simulink model "tilt_rotor_drone_controller"  (R2020b)
settings: Solver=VariableStepAuto  StartTime=0.0  StopTime=10.0  RelTol=1e-3
values from neighbouring files (symbols this model uses):
  acceleration_bc = zeros(size(trajectory))    [run_sim.m]
  b = 20    [run_sim.m]
  d = 0.5    [run_sim.m]
  gamma = [alpha; beta]    [run_sim.m]
  inertia = [0.0092, 0, 0 ... (first row only)    [run_sim.m]    (also in symbolic_equations.m = [Ixx, 0, 0)
  J_TP = 0.5    [run_sim.m]
  K_attitude = lqr(A_attitude, B_attitude, Q_a, R_a)    [run_sim.m]
  K_gamma = lqr(A_gamma, B_gamma, Q_g, R_g)    [run_sim.m]
  K_gamma_plane = lqr(A_gamma_plane, B_gamma_plane, Q_g_p, R_g_p)    [run_sim.m]
  K_position = lqr(A_position, B_position, Q_p, R_p)    [run_sim.m]
  k_r_attitude = -inv(C_attitude/(A_attitude-B_attitude*K_attitude)*B_attitude)    [run_sim.m]
  k_r_gamma = -inv(C_gamma/(A_gamma-B_gamma*K_gamma)*B_gamma)    [run_sim.m]
  k_r_gamma_plane = -inv(C_gamma_plane/(A_gamma_plane-B_gamma_plane*K_gamma_plane)*B_gamma_plane)    [run_sim.m]
  k_r_position = -inv(C_position/(A_position-B_position*K_position)*B_position)    [run_sim.m]
  k_r_thrust = -inv(C_thrust/(A_thrust-B_thrust*K_thrust)*B_thrust)    [run_sim.m]
  k_r_thrust_plane = -inv(C_thrust_plane/(A_thrust_plane-B_thrust_plane*K_thrust_plane)*B_thrust_plane)    [run_sim.m]
  K_thrust = lqr(A_thrust, B_thrust, Q_t, R_t)    [run_sim.m]
  K_thrust_plane = lqr(A_thrust_plane, B_thrust_plane, Q_t_p, R_t_p)    [run_sim.m]
  l_a = 0    [run_sim.m]
  l_l = 0.154    [run_sim.m]
  l_s = 0.19    [run_sim.m]
  lambda = 0.01    [run_sim.m]
  m = 0.736    [run_sim.m]
  mass = [0.736, 0, 0 ... (first row only)    [run_sim.m]    (also in symbolic_equations.m = m*eye(3))
  rho = 1.1455    [run_sim.m]
  trajectory_time = [1;1.1]    [run_sim.m]
  velocity_bc = zeros(size(trajectory))    [run_sim.m]
  wing_area = 0.000124    [run_sim.m]
undefined symbols (not defined in the file or in its folder): trajectory
libraries: simulink x2, robotcorelib x1
settings Model: OrderedModelArguments=off  Creator=Peter Guglielmino  LastModifiedBy=Peter Guglielmino

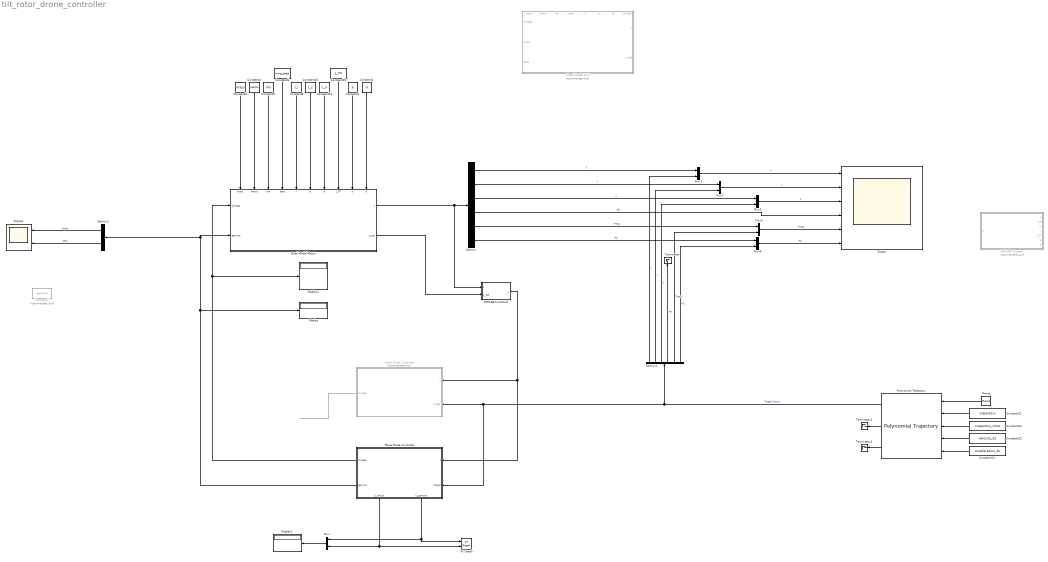
== system tilt_rotor_drone_controller ==
  Constant1 : Constant  Value=b
  Constant10 : Constant  Value=l_s
  Constant13 : Constant  Value=l_a
  Constant2 : Constant  Value=d
  Constant20 : Constant  Value=J_TP
  Constant21 : Constant  Value=trajectory
  Constant22 : Constant  Value=trajectory_time
  Constant23 : Constant  Value=velocity_bc
  Constant24 : Constant  Value=acceleration_bc
  Constant3 : Constant  Value=mass
  Constant4 : Constant  Value=inertia
  Constant5 : Constant  Value=rho
  Constant6 : Constant  Value=wing_area
  Constant7 : Constant  Commented=on  Value=gamma
  Constant8 : Constant  Value=l_l
  Demux : Demux  Outputs=6
  Demux1 : Demux  Outputs=6
  Demux2 : Demux  Outputs=2
  Display : Display
  Display1 : Display
  Display2 : Display
  MATLAB Function : MATLAB Function  Commented=on  TreatAsAtomicUnit=on
  MATLAB Function5 : MATLAB Function  TreatAsAtomicUnit=on
  Mux{,1..5} (6 alike) : Mux  Inputs=2
  Plane Mode Controller : Subsystem
      settings: PortSchema="{\"entries\":[{\"content\":{\"sides\":[{\"content\":{\"connectorIds\":[\"In1\",\"In2\"]},\"type\":\"ConnectorPlacement.EquallySpacedRectSide\",\"uuid\":\"6f4ab3d3-eac6-4fe7-882a-bf2bc23f7ce9\"},{\"content\":{\"connectorIds\":[\"Out1\",\"Out2\"],\"side\":\"RIGHT\"},\"type\":\"ConnectorPlacement.EquallySpacedRectSide\",\"uuid\":\"57ff6c0b-41a8-4a8e-965c-38eb7a1958d7\"},{\"content\":{\"connectorIds\":[],\"side\":\"TOP\"},\"type\":\"ConnectorPlacement.EquallySpacedRectSide\",\"uuid\":\"d6c000f9-9176-43aa-bed6-709b95eb6172\"},{\"content\":{\"connectorIds\":[\"Out3\",\"Out4\"],\"side\":\"BOTTOM\"},\"type\":\"ConnectorPlacement.EquallySpacedRectSide\",\"uuid\":\"a246838b-1dc3-4a22-8023-67a4513b6f5e\"},{\"content\":{\"connectorIds\":[],\"side\":\"HIDDEN\"},\"type\":\"ConnectorPlacement.EquallySpacedRectSide\",\"uuid\":\"9f6f7c1c-aac2-49da-b94c-aa51beb3e11f\"}]},\"type\":\"ConnectorPlacement.EquallySpacedConnector\",\"uuid\":\"622dfaee-5f58-465b-aaa6-50ca0be46197\"}],\"packageUris\":[\"http://schema.mathworks.com/mf0/Connector/R2020b\"],\"version\":\"1.0\"}"
  Polynomial Trajectory : robotcorelib/Polynomial Trajectory  WaypointSource=External  Waypoints=[ 0, 2, 1, 5, 0; -1, 3, 1, 4, 4 ]  TimePoints=[ 0, 1, 2, 3, 4 ]  TimeInterval=[ 1, 4 ]  Method=Quintic Polynomial  ParameterSource=External  VelocityBoundaryCondition=zeros( 2, 5 )  AccelerationBoundaryCondition=zeros( 2, 5 )  SimulateUsing=Interpreted execution
  Quad Mode Controller : Subsystem  Commented=on
  Quad Model F+T : Subsystem  Commented=on
      settings: PortSchema="{\"entries\":[{\"content\":{\"sides\":[{\"content\":{\"connectorIds\":[\"In1\",\"In2\",\"In3\"]},\"type\":\"ConnectorPlacement.EquallySpacedRectSide\",\"uuid\":\"ad073603-3175-40d7-badf-d0e8bcd3f5ed\"},{\"content\":{\"connectorIds\":[\"Out1\",\"Out2\"],\"side\":\"RIGHT\"},\"type\":\"ConnectorPlacement.EquallySpacedRectSide\",\"uuid\":\"d906b516-fe23-4864-8189-1266b65c4bc1\"},{\"content\":{\"connectorIds\":[\"In4\",\"In5\",\"In6\",\"In7\",\"In8\",\"In9\",\"In10\",\"In11\"],\"side\":\"TOP\"},\"type\":\"ConnectorPlacement.EquallySpacedRectSide\",\"uuid\":\"46f69527-661d-433d-ab7a-9aa34cf6966e\"},{\"content\":{\"connectorIds\":[],\"side\":\"HIDDEN\"},\"type\":\"ConnectorPlacement.EquallySpacedRectSide\",\"uuid\":\"d94401f6-fb94-4af8-bf07-62f60ce614d3\"}]},\"type\":\"ConnectorPlacement.EquallySpacedConnector\",\"uuid\":\"9f65350c-1024-4a5e-93be-50f079c0cc08\"}],\"packageUris\":[\"http://schema.mathworks.com/mf0/Connector/R2020b\"],\"version\":\"1.0\"}"
  Quad Model Matrix : Subsystem
      settings: PortSchema="{\"entries\":[{\"content\":{\"sides\":[{\"content\":{\"connectorIds\":[\"In1\",\"In2\"]},\"type\":\"ConnectorPlacement.EquallySpacedRectSide\",\"uuid\":\"7ecde903-2331-4a53-a39c-16ea178ab1ed\"},{\"content\":{\"connectorIds\":[\"Out1\",\"Out2\"],\"side\":\"RIGHT\"},\"type\":\"ConnectorPlacement.EquallySpacedRectSide\",\"uuid\":\"6c8afcf7-f2a3-489f-9b49-f136426d5410\"},{\"content\":{\"connectorIds\":[\"In3\",\"In4\",\"In5\",\"In6\",\"In7\",\"In8\",\"In9\",\"In10\",\"In11\",\"In12\"],\"side\":\"TOP\"},\"type\":\"ConnectorPlacement.EquallySpacedRectSide\",\"uuid\":\"0140aa1b-fbb5-4f49-aa9b-68a16b457c8d\"},{\"content\":{\"connectorIds\":[],\"side\":\"HIDDEN\"},\"type\":\"ConnectorPlacement.EquallySpacedRectSide\",\"uuid\":\"90be69ad-385b-43a9-9593-2c36f7e28e6a\"}]},\"type\":\"ConnectorPlacement.EquallySpacedConnector\",\"uuid\":\"53a680ce-3107-460b-8e4c-bf9b774de8db\"}],\"packageUris\":[\"http://schema.mathworks.com/mf0/Connector/R2020b\"],\"version\":\"1.0\"}"
  Ramp : simulink/Sources/Ramp  slope=0.5  start=0  InitialOutput=0
  Scope : Scope  NumInputPorts=6
  Scope1 : Scope  NumInputPorts=2
  Terminator : Terminator
  Terminator1 : Terminator
  Terminator2 : Terminator
  XY Graph : simulink/Sinks/XY Graph  xmin=-1  xmax=1  ymin=-1  ymax=1  st=-1
  wires:
  Quad Model Matrix/1(s) -> MATLAB Function5/1(s), Demux/1
  Demux/1 -> Mux1/1  "X"
  Demux/2 -> Mux2/1  "Y"
  Demux/3 -> Mux3/1  "Z"
  Demux/4 -> Scope/4  "Phi"
  Demux/6 -> Mux4/1  "Psi"
  Quad Model Matrix/2(s_dot) -> MATLAB Function5/2(s_dot)
  Demux1/6 -> Mux4/2  "Psi"
  Demux1/1 -> Mux1/2  "X"
  Demux1/3 -> Mux3/2  "Z"
  Demux1/2 -> Mux2/2  "Y"
  Mux1/1 -> Scope/1  "X"
  Mux2/1 -> Scope/2  "Y"
  Mux3/1 -> Scope/3  "Z"
  Mux4/1 -> Scope/6  "Psi"
  Constant3/1 -> Quad Model Matrix/3(mass)
  Constant4/1 -> Quad Model Matrix/4(inertia)
  Constant5/1 -> Quad Model Matrix/5(rho)
  Constant6/1 -> Quad Model Matrix/6(area)
  Constant8/1 -> Quad Model Matrix/7(ll)
  Constant10/1 -> Quad Model Matrix/8(ls)
  Constant13/1 -> Quad Model Matrix/9(la)
  Constant20/1 -> Quad Model Matrix/10(J_TP)
  Demux1/5 -> Mux5/2  "Theta"
  Demux/5 -> Mux5/1  "Theta"
  Mux5/1 -> Scope/5  "Theta"
  Constant1/1 -> Quad Model Matrix/11(b)
  Constant2/1 -> Quad Model Matrix/12(d)
  Polynomial Trajectory/1 -> Plane Mode Controller/2(Target), Quad Mode Controller/2(Target), Demux1/1  "Target Vector"
  Ramp/1 -> Polynomial Trajectory/1
  Constant22/1 -> Polynomial Trajectory/3
  Constant21/1 -> Polynomial Trajectory/2
  Constant23/1 -> Polynomial Trajectory/4
  Constant24/1 -> Polynomial Trajectory/5
  Demux1/4 -> Terminator/1  "Phi"
  Polynomial Trajectory/2 -> Terminator1/1
  Polynomial Trajectory/3 -> Terminator2/1
  MATLAB Function5/1(y) -> Plane Mode Controller/1(s), Quad Mode Controller/1(s)
  Demux2/1 -> Scope1/1  "alpha"
  Demux2/2 -> Scope1/2  "beta"
  Plane Mode Controller/2(gamma) -> Demux2/1, Quad Model Matrix/2(gamma), Display/1
  Plane Mode Controller/1(Omega) -> Display2/1, Quad Model Matrix/1(Omega)
  Quad Mode Controller/1(Omega) -> ?
  Plane Mode Controller/3(U_gamma) -> Mux/1, XY Graph/1
  Plane Mode Controller/4(U_thrust) -> XY Graph/2, Mux/2
  Mux/1 -> Display1/1

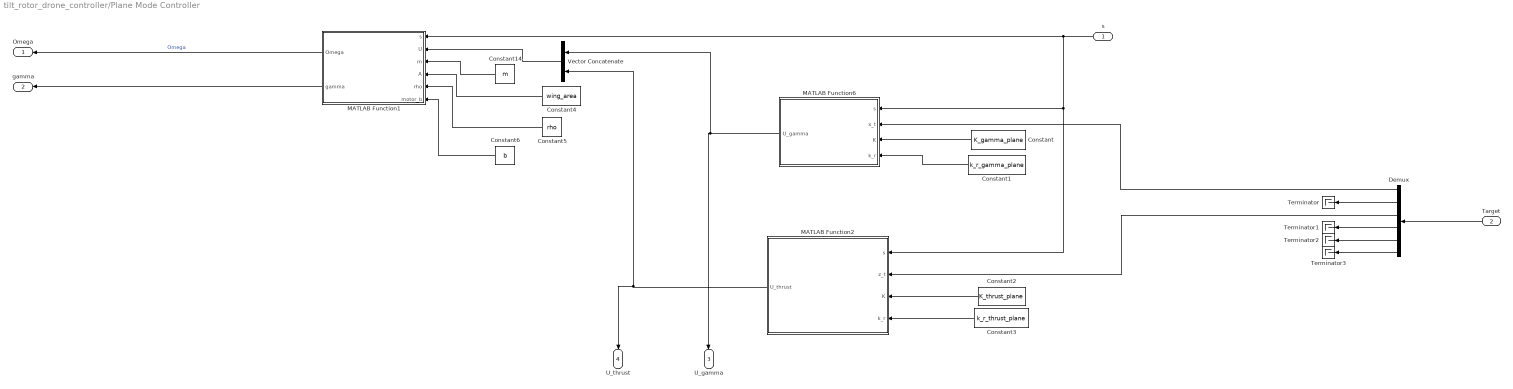
== system tilt_rotor_drone_controller/Plane Mode Controller ==
  s : Inport
  Target : Inport  Port=2
  Constant : Constant  Value=K_gamma_plane
  Constant1 : Constant  Value=k_r_gamma_plane
  Constant14 : Constant  Value=m
  Constant2 : Constant  Value=K_thrust_plane
  Constant3 : Constant  Value=k_r_thrust_plane
  Constant4 : Constant  Value=wing_area
  Constant5 : Constant  Value=rho
  Constant6 : Constant  Value=b
  Demux : Demux  Outputs=6
  MATLAB Function1 : MATLAB Function  TreatAsAtomicUnit=on
  MATLAB Function2 : MATLAB Function  TreatAsAtomicUnit=on
  MATLAB Function6 : MATLAB Function  TreatAsAtomicUnit=on
  Terminator{,1..3} (4 alike) : Terminator
  Vector Concatenate : Concatenate
  Omega : Outport
  gamma : Outport  Port=2
  U_gamma : Outport  Port=3
  U_thrust : Outport  Port=4
  wires:
  Demux/3 -> MATLAB Function2/2(z_t)
  s/1 -> MATLAB Function2/1(s), MATLAB Function6/1(s), MATLAB Function1/1(s)
  MATLAB Function1/1(Omega) -> Omega/1  "Omega"
  Vector Concatenate/1 -> MATLAB Function1/2(U)
  Constant14/1 -> MATLAB Function1/3(m)
  MATLAB Function2/1(U_thrust) -> U_thrust/1, Vector Concatenate/2
  MATLAB Function1/2(gamma) -> gamma/1
  Constant2/1 -> MATLAB Function2/3(K)
  Constant3/1 -> MATLAB Function2/4(k_r)
  Constant/1 -> MATLAB Function6/3(K)
  Constant1/1 -> MATLAB Function6/4(k_r)
  Constant4/1 -> MATLAB Function1/4(A)
  Constant5/1 -> MATLAB Function1/5(rho)
  MATLAB Function6/1(U_gamma) -> Vector Concatenate/1, U_gamma/1
  Constant6/1 -> MATLAB Function1/6(motor_b)
  Target/1 -> Demux/1
  Demux/1 -> MATLAB Function6/2(x_t)
  Demux/2 -> Terminator/1
  Demux/4 -> Terminator1/1
  Demux/5 -> Terminator2/1
  Demux/6 -> Terminator3/1

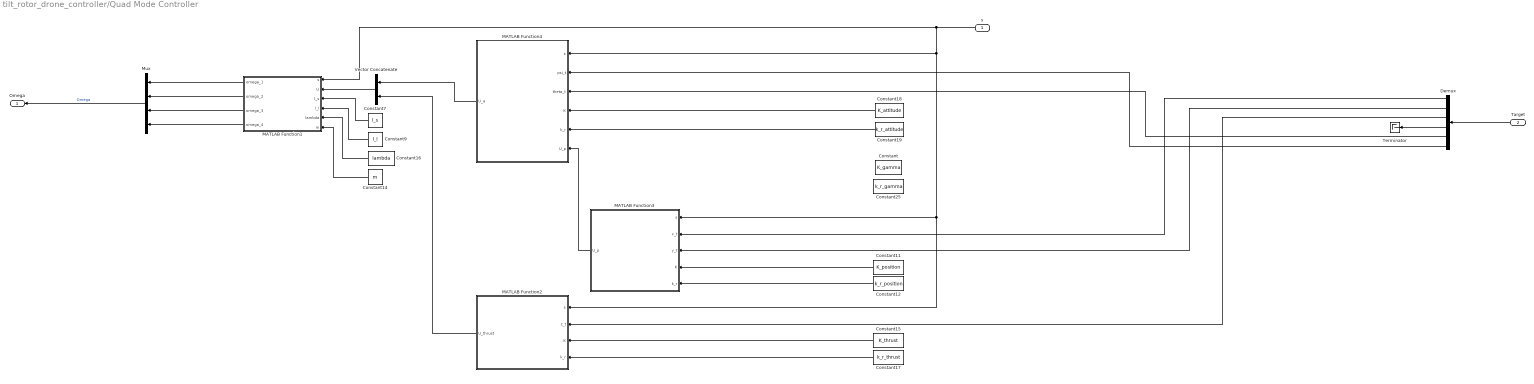
== system tilt_rotor_drone_controller/Quad Mode Controller ==
  s : Inport
  Target : Inport  Port=2
  Constant : Constant  Value=K_gamma
  Constant11 : Constant  Value=K_position
  Constant12 : Constant  Value=k_r_position
  Constant14 : Constant  Value=m
  Constant15 : Constant  Value=K_thrust
  Constant16 : Constant  Value=lambda
  Constant17 : Constant  Value=k_r_thrust
  Constant18 : Constant  Value=K_attitude
  Constant19 : Constant  Value=k_r_attitude
  Constant25 : Constant  Value=k_r_gamma
  Constant7 : Constant  Value=l_s
  Constant9 : Constant  Value=l_l
  Demux : Demux  Outputs=6
  MATLAB Function1 : MATLAB Function  TreatAsAtomicUnit=on
  MATLAB Function2 : MATLAB Function  TreatAsAtomicUnit=on
  MATLAB Function3 : MATLAB Function  TreatAsAtomicUnit=on
  MATLAB Function4 : MATLAB Function  TreatAsAtomicUnit=on
  Mux : Mux
  Terminator : Terminator
  Vector Concatenate : Concatenate
  Omega : Outport
  wires:
  Constant11/1 -> MATLAB Function3/4(K)
  MATLAB Function1/3(omega_3) -> Mux/3
  MATLAB Function1/1(omega_1) -> Mux/1
  s/1 -> MATLAB Function2/1(s), MATLAB Function3/1(s), MATLAB Function4/1(s), MATLAB Function1/1(s)
  MATLAB Function4/1(U_a) -> Vector Concatenate/1
  MATLAB Function1/2(omega_2) -> Mux/2
  MATLAB Function2/1(U_thrust) -> Vector Concatenate/2
  Constant17/1 -> MATLAB Function2/4(k_r)
  Constant16/1 -> MATLAB Function1/5(lambda)
  Constant14/1 -> MATLAB Function1/6(m)
  MATLAB Function1/4(omega_4) -> Mux/4
  MATLAB Function3/1(U_p) -> MATLAB Function4/6(U_p)
  Constant7/1 -> MATLAB Function1/3(l_s)
  Constant9/1 -> MATLAB Function1/4(l_l)
  Demux/6 -> MATLAB Function4/2(psi_t)
  Constant12/1 -> MATLAB Function3/5(k_r)
  Constant19/1 -> MATLAB Function4/5(k_r)
  Vector Concatenate/1 -> MATLAB Function1/2(U)
  Demux/5 -> MATLAB Function4/3(theta_t)
  Constant15/1 -> MATLAB Function2/3(K)
  Constant18/1 -> MATLAB Function4/4(K)
  Demux/1 -> MATLAB Function3/2(x_t)
  Mux/1 -> Omega/1  "Omega"
  Demux/2 -> MATLAB Function3/3(y_t)
  Demux/3 -> MATLAB Function2/2(z_t)
  Demux/4 -> Terminator/1
  Target/1 -> Demux/1

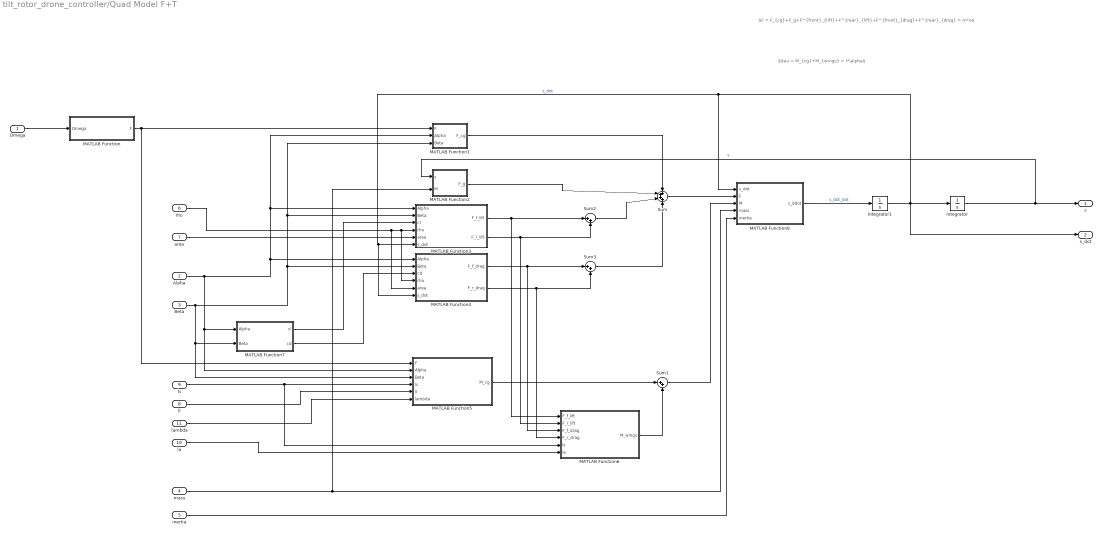
== system tilt_rotor_drone_controller/Quad Model F+T ==
  note: $\tau = M_{cg}+M_{wings} = I*\alpha$
  note: $F = F_{cg}+F_g+F^{front}_{lift}+F^{rear}_{lift}+F^{front}_{drag}+F^{rear}_{drag} = m*a$
  Omega : Inport
  Alpha : Inport  Port=2
  Beta : Inport  Port=3
  mass : Inport  Port=4
  inertia : Inport  Port=5
  rho : Inport  Port=6
  area : Inport  Port=7
  ll : Inport  Port=8
  ls : Inport  Port=9
  la : Inport  Port=10
  lambda : Inport  Port=11
  Integrator : Integrator
  Integrator1 : Integrator
  MATLAB Function : MATLAB Function  TreatAsAtomicUnit=on
  MATLAB Function1 : MATLAB Function  TreatAsAtomicUnit=on
  MATLAB Function2 : MATLAB Function  TreatAsAtomicUnit=on
  MATLAB Function3 : MATLAB Function  TreatAsAtomicUnit=on
  MATLAB Function4 : MATLAB Function  TreatAsAtomicUnit=on
  MATLAB Function5 : MATLAB Function  TreatAsAtomicUnit=on
  MATLAB Function6 : MATLAB Function  TreatAsAtomicUnit=on
  MATLAB Function7 : MATLAB Function  TreatAsAtomicUnit=on
  MATLAB Function8 : MATLAB Function  TreatAsAtomicUnit=on
  Sum : Sum  Inputs=++++
  Sum1 : Sum  Inputs=|++
  Sum2 : Sum  Inputs=|++
  Sum3 : Sum  Inputs=|++
  s : Outport
  s_dot : Outport  Port=2
  wires:
  MATLAB Function/1(F) -> MATLAB Function1/1(F), MATLAB Function5/1(F)
  MATLAB Function7/2(cd) -> MATLAB Function4/3(cd)
  MATLAB Function7/1(cl) -> MATLAB Function3/3(cl)
  inertia/1 -> MATLAB Function8/5(inertia)
  mass/1 -> MATLAB Function2/2(M), MATLAB Function8/4(mass)
  Sum1/1 -> MATLAB Function8/3(M)
  Sum/1 -> MATLAB Function8/2(F)
  la/1 -> MATLAB Function6/6(la)
  MATLAB Function4/2(F_r_drag) -> Sum3/2, MATLAB Function6/4(F_r_drag)
  MATLAB Function4/1(F_f_drag) -> Sum3/1, MATLAB Function6/3(F_f_drag)
  MATLAB Function3/2(F_r_lift) -> Sum2/2, MATLAB Function6/2(F_r_lift)
  MATLAB Function3/1(F_f_lift) -> Sum2/1, MATLAB Function6/1(F_f_lift)
  Sum3/1 -> Sum/4
  Sum2/1 -> Sum/3
  lambda/1 -> MATLAB Function5/6(lambda)
  ll/1 -> MATLAB Function5/5(ll)
  ls/1 -> MATLAB Function5/4(ls), MATLAB Function6/5(ls)
  area/1 -> MATLAB Function3/5(area)
  rho/1 -> MATLAB Function3/4(rho), MATLAB Function4/4(rho), MATLAB Function4/5(area)
  Beta/1 -> MATLAB Function3/2(Beta), MATLAB Function1/3(Beta), MATLAB Function4/2(Beta), MATLAB Function7/2(Beta), MATLAB Function5/3(Beta)
  Alpha/1 -> MATLAB Function4/1(Alpha), MATLAB Function3/1(Alpha), MATLAB Function1/2(Alpha), MATLAB Function7/1(Alpha), MATLAB Function5/2(Alpha)
  MATLAB Function8/1(s_ddot) -> Integrator1/1  "s_dot_dot"
  MATLAB Function6/1(M_wings) -> Sum1/2
  MATLAB Function5/1(M_cg) -> Sum1/1
  MATLAB Function2/1(F_g) -> Sum/2
  MATLAB Function1/1(F_cg) -> Sum/1
  Omega/1 -> MATLAB Function/1(Omega)
  Integrator1/1 -> s_dot/1, Integrator/1, MATLAB Function8/1(s_dot), MATLAB Function3/6(s_dot), MATLAB Function4/6(s_dot)  "s_dot"
  Integrator/1 -> s/1, MATLAB Function2/1(s)  "s"

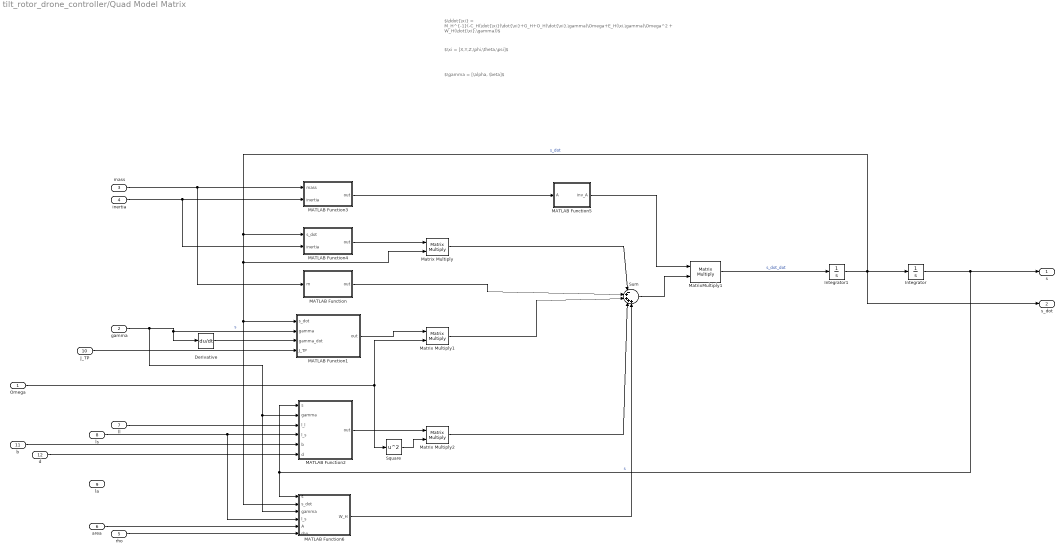
== system tilt_rotor_drone_controller/Quad Model Matrix ==
  note: $\ddot{\xi} = M_H^{-1}(-C_H(\dot{\xi})\dot{\xi}+G_H+O_H(\dot{\xi},\gamma)\Omega+E_H(\xi,\gamma)\Omega^2 + W_H(\dot{\xi},\gamma))$
  note: $\xi = [X,Y,Z,\phi,\theta,\psi]$
  note: $\gamma = [\alpha, \beta]$
  Omega : Inport  PortDimensions=[4,1]
  gamma : Inport  Port=2  PortDimensions=[2 1]
  mass : Inport  Port=3
  inertia : Inport  Port=4
  rho : Inport  Port=5
  area : Inport  Port=6
  ll : Inport  Port=7
  ls : Inport  Port=8
  la : Inport  Port=9
  J_TP : Inport  Port=10
  b : Inport  Port=11
  d : Inport  Port=12
  Derivative : Derivative
  Integrator : Integrator
  Integrator1 : Integrator
  MATLAB Function : MATLAB Function  TreatAsAtomicUnit=on
  MATLAB Function1 : MATLAB Function  TreatAsAtomicUnit=on
  MATLAB Function2 : MATLAB Function  TreatAsAtomicUnit=on
  MATLAB Function3 : MATLAB Function  TreatAsAtomicUnit=on
  MATLAB Function4 : MATLAB Function  TreatAsAtomicUnit=on
  MATLAB Function5 : MATLAB Function  TreatAsAtomicUnit=on
  MATLAB Function6 : MATLAB Function  TreatAsAtomicUnit=on
  Matrix Multiply : Product  Multiplication=Matrix(*)
  Matrix Multiply1 : Product  Multiplication=Matrix(*)
  Matrix Multiply2 : Product  Multiplication=Matrix(*)
  MatrixMultiply1 : Product  Multiplication=Matrix(*)
  Square : Math  Operator=square  SaturateOnIntegerOverflow=on
  Sum : Sum  Inputs=|-++++
  s : Outport
  s_dot : Outport  Port=2
  wires:
  Integrator/1 -> MATLAB Function2/1(s), MATLAB Function6/1(s), s/1  "s"
  Integrator1/1 -> s_dot/1, MATLAB Function4/1(s_dot), Matrix Multiply/2, MATLAB Function6/2(s_dot), MATLAB Function1/1(s_dot), Integrator/1  "s_dot"
  MatrixMultiply1/1 -> Integrator1/1  "s_dot_dot"
  MATLAB Function/1(out) -> Sum/2
  Matrix Multiply/1 -> Sum/1
  Sum/1 -> MatrixMultiply1/2
  MATLAB Function1/1(out) -> Matrix Multiply1/1
  Matrix Multiply1/1 -> Sum/3
  MATLAB Function2/1(out) -> Matrix Multiply2/1
  Matrix Multiply2/1 -> Sum/4
  mass/1 -> MATLAB Function/1(m), MATLAB Function3/1(mass)
  inertia/1 -> MATLAB Function4/2(inertia), MATLAB Function3/2(inertia)
  ll/1 -> MATLAB Function2/3(l_l)
  ls/1 -> MATLAB Function6/4(l_s), MATLAB Function2/4(l_s)
  b/1 -> MATLAB Function2/5(b)
  d/1 -> MATLAB Function2/6(d)
  J_TP/1 -> MATLAB Function1/4(J_TP)
  MATLAB Function4/1(out) -> Matrix Multiply/1
  Square/1 -> Matrix Multiply2/2
  Omega/1 -> Matrix Multiply1/2, Square/1
  MATLAB Function3/1(out) -> MATLAB Function5/1(A)
  MATLAB Function5/1(inv_A) -> MatrixMultiply1/1
  gamma/1 -> MATLAB Function6/3(gamma), MATLAB Function2/2(gamma), MATLAB Function1/2(gamma), Derivative/1  "s"
  area/1 -> MATLAB Function6/5(A)
  rho/1 -> MATLAB Function6/6(rho)
  MATLAB Function6/1(W_H) -> Sum/5
  Derivative/1 -> MATLAB Function1/3(gamma_dot)

== matlab function tilt_rotor_drone_controller/Quad Mode Controller/MATLAB Function2 ==
  data: s input; z_t input; K input size=[1 2]; k_r input size=1; U_thrust output
function U_thrust = thrust_control(s, z_t, K, k_r)

% s = [x, dx, y, dy, z, dz, phi, p, theta, q, psi, r]

x = s(5:6);
x_d = [z_t; 0];

C = [1,0];
r = C*x_d;

U_thrust = -K*x + k_r*r;

== matlab function tilt_rotor_drone_controller/Quad Mode Controller/MATLAB Function3 ==
  data: s input; U_p output; x_t input; y_t input; K input size=[2 4]; k_r input size=[2 2]
function U_p = position_control(s, x_t, y_t, K, k_r)

% s = [x, dx, y, dy, z, dz, phi, p, theta, q, psi, r]

x = s(1:4);
x_d = [x_t;0;y_t;0];
  
C = [1,0,0,0;
     0,0,1,0];

r = C*x_d;
U_p = -K*x + k_r*r;

== matlab function tilt_rotor_drone_controller/Quad Mode Controller/MATLAB Function4 ==
  data: s input; psi_t input; theta_t input; U_a output; K input size=[3 6]; k_r input size=[3 3]; U_p input
function U_a  = attitude_control(s, psi_t, theta_t, K, k_r, U_p)

% s = [x, dx, y, dy, z, dz, !phi, p, theta, q, psi, r!]
% U_p = [U_x, U_y]
% U_x = (cos(phi)*sin(theta)*cos(psi) + sin(phi)*sin(psi))/(cos(phi)*cos(theta))
% U_y = (cos(phi)*sin(theta)*sin(psi) - sin(phi)*cos(psi))/(cos(phi)*cos(theta))
% theta = atan2(U_y + U_x*tan(psi),sin(psi)-cos(psi)^2)
% phi = atan2(U_x*cos(theta)-sin(theta)*cos(psi),sin(psi))

% alpha = 0;
% beta = 0;


x = s(7:12);

U_x = U_p(1);
U_y = U_p(2);

psi = x(5);
Kappa = U_x^2 + U_y^2;

if (U_x^2 + U_y^2) == 0
    phi = 0;
else
    phi = asin(sqrt(Kappa/((1+Kappa)*(U_x^2+U_y^2))) * (U_x*sin(psi) - U_y*cos(psi)));
end

s = sign(U_y*sin(psi) + U_x*cos(psi));
if abs(1/(cos(phi)*sqrt(1+Kappa))) > 1
    theta = s*acos(sign(1/(cos(phi)*sqrt(1+Kappa))));
else
    theta = s*acos(1/(cos(phi)*sqrt(1+Kappa)));
end

x_d = [phi; 0; theta + theta_t; 0; psi_t; 0];
 
C = [1,0,0,0,0,0;
     0,0,1,0,0,0;
     0,0,0,0,1,0];
 
r = C*x_d;
U_a = -K*x + k_r*r;

== matlab function tilt_rotor_drone_controller/MATLAB Function5 ==
  data: s input; y output; s_dot input
function y = mixer(s, s_dot)

x = [s(1);s_dot(1);s(2);s_dot(2);s(3);s_dot(3);s(4);s_dot(4);s(5);s_dot(5);s(6);s_dot(6)];

y = x;

== matlab function tilt_rotor_drone_controller/Quad Model Matrix/MATLAB Function6 ==
  data: s input size=[6 1]; s_dot input size=[6 1]; W_H output size=[6 1]; gamma input size=[2 1]; l_s input size=1; A input size=1; rho input size=1
function W_H = W_H(s, s_dot, gamma, l_s, A, rho)
% s_dot = [dx, dy, dz, p, q, r]

v = [s_dot(1); 0; s_dot(3)]; % wind velocity ignoring y
wind_vel = norm(v)*v;

alpha = gamma(1);
beta = gamma(2);

phi = s(4);
theta = s(5);
psi = s(6);

alpha_matrix = [cos(alpha),  0, sin(alpha);
                    0,       1,      0;
                -sin(alpha), 0, cos(alpha)];
    
beta_matrix = [cos(beta),  0, sin(beta);
                    0,     1,     0;
               -sin(beta), 0, cos(beta)];

alpha_vector = [-sin(alpha); 0; -cos(alpha)];
beta_vector = [-sin(beta); 0; -cos(beta)];


R = [cos(psi)*cos(theta), -sin(psi)*cos(phi) + cos(psi)*sin(theta)*sin(phi), sin(psi)*sin(phi) + cos(psi)*sin(theta)*cos(phi);
     sin(psi)*cos(theta), cos(psi)*cos(phi) + sin(psi)*sin(theta)*sin(phi), -cos(psi)*sin(phi) + sin(psi)*sin(theta)*cos(phi);
     -sin(theta), cos(theta)*sin(phi), cos(theta)*cos(phi)];
 
T = [R, zeros(3,3);
     zeros(3,3), eye(3)];

if norm(wind_vel) ~= 0
    attack_angle_front = acosd(dot(wind_vel,alpha_vector)/(norm(wind_vel)*norm(alpha_vector)));
    attack_angle_back  = acosd(dot(wind_vel,beta_vector)/(norm(wind_vel)*norm(beta_vector)));
    
    c_la = getLiftCoef(attack_angle_front);
    c_lb = getLiftCoef(attack_angle_back);
    c_da = getDragCoef(attack_angle_front);
    c_db = getDragCoef(attack_angle_back);
else
    c_la = 0;
    c_lb = 0;
    c_da = 0;
    c_db = 0;
end

L_pba = alpha_matrix * [1;0;0] * c_la*rho*A * norm(wind_vel);
L_pbb = beta_matrix * [1;0;0] * c_lb*rho*A * norm(wind_vel);
L_pb = L_pba + L_pbb;
L_tb = cross([l_s;0;0], L_pba) + cross([-l_s;0;0], L_pbb);

L_H = T*[L_pb;
         L_tb];
     
D_pba = alpha_matrix * [0;0;1] * c_da*rho*A * norm(wind_vel);
D_pbb = beta_matrix * [0;0;1] * c_db*rho*A * norm(wind_vel);
D_pb = D_pba + D_pbb;
D_tb = cross([l_s;0;0], D_pba) + cross([-l_s;0;0], D_pbb);

D_H = T*[D_pb;
         D_tb];

W_H = L_H + D_H;
end


function c_l = getLiftCoef(x)
    if x > 0 && x < 80
        c_l = -3E-10*x^6 + 7E-08*x^5 - 6E-06*x^4 + 0.0002*x^3 - 0.0042*x^2 + 0.0495*x + 0.0485;
    else
        c_l = 0;
    end
end

function c_d = getDragCoef(x)
    if x > 0 && x < 80
        c_d = 4E-09*x^5 - 8E-07*x^4 + 4E-05*x^3 - 0.0006*x^2 + 0.004*x + 0.0403;
    else
        c_d = 0;
    end
end

== matlab function tilt_rotor_drone_controller/Plane Mode Controller/MATLAB Function1 ==
  data: s input; U input size=[2 1]; Omega output size=[4 1]; m input; gamma output; A input; rho input; motor_b input
function [Omega, gamma]= U_to_Omega(s, U, m, A, rho, motor_b)
% s = [x, dx, y, dy, z, dz, phi, p, theta, q, psi, r]
% U = [U_G, U_T]

U_G = U(1);
U_T = U(2);

g = 9.8;

control_vector = [U_G; U_T];

if norm(control_vector) == 0
    control_angle = 0;
else
    control_angle = -pi/2 + atan2(-control_vector(2),control_vector(1));
end

thrust_value = norm(control_vector);

control_angle = min(max(control_angle, -pi/2), pi/2);

% v = [s(2); 0; s(6)]; % wind velocity ignoring y
% v_w = norm(v)*v;
% 
% alpha_old = -pi/3;
% 
% alpha_vector = [-sin(alpha_old); 0; -cos(alpha_old)];
% 
% phi = s(7);
% theta = s(9);
% psi = s(11);
% 
% K1 = cos(psi)*cos(theta);
% K2 = sin(phi)*sin(psi) + cos(phi)*cos(psi)*sin(theta);
% 
% K3 = sin(theta);
% K4 = cos(phi)*cos(theta);
% 
% if norm(v_w) ~= 0
%     attack_angle_front = acosd(dot(v_w,alpha_vector)/(norm(v_w)*norm(alpha_vector)));
%     
%     c_la = getLiftCoef(attack_angle_front);
%     c_da = getDragCoef(attack_angle_front);
% else
%     c_la = 0;
%     c_da = 0;
% end

% a = K4;
% b = K3;
% c = -m*(U_G - g)/(2*A*rho*norm(v_w)*c_la);
% if c == Inf
%     alpha = alpha_old;
% else
%     d = sqrt(-1*(c^2 - b^2 - a^2));
%     alpha = atan((b*d + a*c)/(b*c - a*d));
% end

% if norm(v_w) ~= 0
%     alpha = alpha_old;
% else
% %     alpha = asin(-m*(U_G - g)/(2*A*rho*norm(v_w)*c_la));
%     alpha = alpha_old;
% end

% omega_1_sqr = -U_T*m/(8*motor_b*(sin(alpha)*K1 + cos(alpha)*K2));
% omega_1_sqr = -((U_T*m + 2*A*rho*norm(v_w)*c_la*cos(alpha) - 2*A*rho*norm(v_w)*c_da*sin(alpha))/(8*motor_b));

alpha = control_angle;
omega_1_sqr = thrust_value;

if (omega_1_sqr > 0)
    omega_1 = sqrt(omega_1_sqr);
else
    omega_1 = 0;
end

gamma = [alpha; alpha];
Omega = [omega_1; omega_1; omega_1; omega_1];

end

function c_l = getLiftCoef(x)
    c_l = -3E-10*x^6 + 7E-08*x^5 - 6E-06*x^4 + 0.0002*x^3 - 0.0042*x^2 + 0.0495*x + 0.0485;
end

function c_d = getDragCoef(x)
    c_d = 4E-09*x^5 - 8E-07*x^4 + 4E-05*x^3 - 0.0006*x^2 + 0.004*x + 0.0403;
end

== matlab function tilt_rotor_drone_controller/Quad Model F+T/MATLAB Function ==
  data: Omega input; F output size=[4 1]
function F = Omega_to_F(Omega)

F = eye(4)*Omega;

== matlab function tilt_rotor_drone_controller/Quad Model F+T/MATLAB Function1 ==
  data: F input; F_cg output; Alpha input; Beta input
function F_cg = F_cg(F, Alpha, Beta)
% Force generated from the rotors

F_cg = [-sin(Alpha)*(F(1)+F(2)) - sin(Beta)*(F(3)+F(4));
                            0;
     -cos(Alpha)*(F(1)+F(2)) - cos(Beta)*(F(3)+F(4))];

== matlab function tilt_rotor_drone_controller/Quad Model F+T/MATLAB Function2 ==
  data: s input; M input; F_g output
function F_g = F_g(s, M)
% s = [x, y, z, phi, theta, psi]
theta = s(5);
phi = s(4);
g = 9.8;

rotation = [-sin(theta);
            sin(phi)*cos(theta);
            cos(phi)*cos(theta)];

F_g = M*rotation*g;

== matlab function tilt_rotor_drone_controller/Quad Model F+T/MATLAB Function3 ==
  data: F_f_lift output; Alpha input; Beta input; cl input; rho input; area input; s_dot input; F_r_lift output
function [F_f_lift, F_r_lift] = F_lift(Alpha, Beta, cl, rho, area, s_dot)
% s_dot = [dx, dy, dz, p, q, r]

Ry_a = [cos(Alpha), 0, sin(Alpha);
             0,     1,      0;
        -sin(Alpha), 0, cos(Alpha)];

Ry_b = [cos(Beta), 0, sin(Beta);
             0,     1,      0;
        -sin(Beta), 0, cos(Beta)];

w_hat = [0;0;-1];

v = [s_dot(1);s_dot(2);s_dot(3)];
v_f = dot(Ry_a * w_hat,v);
v_r = dot(Ry_b * w_hat,v);


F_f_lift = Ry_a * [-2*(1/2)*cl(1)*rho*area*v_f^2;0;0];
F_r_lift = Ry_b * [-2*(1/2)*cl(2)*rho*area*v_r^2;0;0];

== matlab function tilt_rotor_drone_controller/Quad Model Matrix/MATLAB Function1 ==
  data: s_dot input; gamma input size=[2 1]; out output size=[6,4]; gamma_dot input size=[2 1]; J_TP input
function out = O_H(s_dot, gamma, gamma_dot, J_TP)

w_b = s_dot(4:6);

alpha = gamma_dot(1);
beta = gamma(2);

alpha_dot = gamma_dot(1);
beta_dot = gamma_dot(2);

alpha_vector = [-sin(alpha); 0; -cos(alpha)];
beta_vector = [-sin(beta); 0; -cos(beta)];

a_vector = cross(w_b, alpha_vector) + cross([0; alpha_dot; 0], alpha_vector);
b_vector = cross(w_b, beta_vector) + cross([0; beta_dot; 0], beta_vector);
four_vector = [a_vector, -a_vector, -b_vector, b_vector];
O_H = [zeros(3,4);  four_vector];

out = J_TP * O_H;

== matlab function tilt_rotor_drone_controller/Quad Model F+T/MATLAB Function4 ==
  data: Alpha input; Beta input; F_f_drag output; cd input; rho input; area input; s_dot input; F_r_drag output
function [F_f_drag, F_r_drag] = F_drag(Alpha, Beta, cd, rho, area, s_dot)
% s_dot = [dx, dy, dz, p, q, r]

Ry_a = [cos(Alpha), 0, sin(Alpha);
             0,     1,      0;
        -sin(Alpha), 0, cos(Alpha)];

Ry_b = [cos(Beta), 0, sin(Beta);
             0,     1,      0;
        -sin(Beta), 0, cos(Beta)];

w_hat = [0;0;-1];

v = [s_dot(1);s_dot(2);s_dot(3)];
v_f = dot(Ry_a * w_hat,v);
v_r = dot(Ry_b * w_hat,v);


F_f_drag = Ry_a * [0;0;2*(1/2)*cd(1)*rho*area*v_f^2];
F_r_drag = Ry_b * [0;0;2*(1/2)*cd(2)*rho*area*v_r^2];

== matlab function tilt_rotor_drone_controller/Quad Model F+T/MATLAB Function5 ==
  data: F input; M_cg output; Alpha input; Beta input; ls input; ll input; lambda input
function M_cg = M_cg(F, Alpha, Beta, ls, ll, lambda)

Ry_a = [cos(Alpha), 0, sin(Alpha);
            0,     1,      0;
        -sin(Alpha), 0, cos(Alpha)];

Ry_b = [cos(Beta), 0, sin(Beta);
            0,     1,      0;
        -sin(Beta), 0, cos(Beta)];

moment_arm_f = [ls, -ls;
                ll, ll;
                lambda, -lambda];
            
moment_arm_r = [ls, -ls;
                -ll, -ll;
                -lambda, lambda];

M_cg = Ry_a * moment_arm_f * [F(1); F(2)] + Ry_b * moment_arm_r * [F(3); F(4)];

== matlab function tilt_rotor_drone_controller/Quad Model F+T/MATLAB Function6 ==
  data: F_f_lift input; M_wings output; F_r_lift input; F_f_drag input; F_r_drag input; ls input; la input
function M_wings = M_wings(F_f_lift, F_r_lift, F_f_drag, F_r_drag, ls, la)

moment_arm_f = [0, 0, 0;
              -la, 0, -ls;
              0, 0, 0];

moment_arm_r = [0, 0, 0;
              -la, 0, ls;
              0, 0, 0];         
          
M_wings = moment_arm_f*(F_f_lift + F_f_drag) + moment_arm_r*(F_r_lift + F_r_drag);

== matlab function tilt_rotor_drone_controller/Quad Model F+T/MATLAB Function7 ==
  data: Alpha input; cl output; Beta input; cd output
function [cl,cd] = lift_and_drag(Alpha, Beta)

% cl = [cl_f; cl_r]
% cd = [cd_f; cd_r]

cl = [Alpha; Alpha];
cd = [Beta; Beta];

== matlab function tilt_rotor_drone_controller/Quad Model F+T/MATLAB Function8 ==
  data: s_dot input; s_ddot output size=[6 1]; F input; M input; mass input; inertia input
function s_ddot = s_ddot(s_dot, F, M, mass, inertia)
% s_dot = [dx, dy, dz, p, q, r]
% 
% R_x = [1, 0, 0;
%      0, cos(s(7)), -sin(s(7));
%      0, sin(s(7)), cos(s(7))];
% 
% R_y = [cos(s(9)), 0, sin(s(9));
%          0,   1,    0;
%        -sin(s(9)), 0, cos(s(9))];
%   
% R_z = [cos(s(11)), -sin(s(11)), 0;
%        sin(s(11)), cos(s(11)),  0;
%          0,     0,    1];
% 
% T = R_x*R_y*R_z;
% 
% E = [1, 0, -sin(theta);
%      0, cos(theta), sin(phi)*cos(theta);
%      0, -sin(theta), cos(phi)*cos(theta)];

V_b = [s_dot(1);s_dot(2);s_dot(3)];
w_b = [s_dot(4);s_dot(5);s_dot(6)]; 


% P_dot = T\V_b;
V_dot = mass\(F-cross(w_b, mass*V_b));
% Q_dot = E\w_b;
w_dot = inertia\(M-cross(w_b, inertia*w_b));



s_ddot = [V_dot(1); V_dot(2); V_dot(3); w_dot(1); w_dot(2); w_dot(3)];

== matlab function tilt_rotor_drone_controller/Plane Mode Controller/MATLAB Function2 ==
  data: s input; z_t input; K input size=[1 2]; k_r input size=1; U_thrust output
function U_thrust = thrust_control(s, z_t, K, k_r)
% s = [x, dx, y, dy, z, dz, phi, p, theta, q, psi, r]

x = s(5:6);
x_d = [z_t; 0];

C = [1, 0];
r = C*x_d;

U_thrust = -K*x + k_r*r;

== matlab function tilt_rotor_drone_controller/Plane Mode Controller/MATLAB Function6 ==
  data: s input size=[12 1]; x_t input; U_gamma output; K input size=[1 2]; k_r input size=1
function U_gamma = gamma_control(s, x_t, K, k_r)
% s = [x, dx, y, dy, z, dz, phi, p, theta, q, psi, r]
% gamma = [I_alpha, alpha, I_beta, beta]

x = s(1:2);
x_d = [x_t; 0];

C = [1, 0];
r = C*x_d;

U_gamma = -K*x + k_r*r;

== matlab function tilt_rotor_drone_controller/Quad Model Matrix/MATLAB Function ==
  data: m input; out output
function out = G_H(m)

G = m*[0;0;9.8];

out = [G;0;0;0];

== matlab function tilt_rotor_drone_controller/Quad Model Matrix/MATLAB Function2 ==
  data: s input; out output; gamma input size=[2 1]; l_l input; l_s input; b input; d input
function out = E_H(s, gamma, l_l, l_s, b, d)


phi = s(4);
theta = s(5);
psi = s(6);

alpha = gamma(1);
beta = gamma(2);

R = [cos(psi)*cos(theta), -sin(psi)*cos(phi) + cos(psi)*sin(theta)*sin(phi), sin(psi)*sin(phi) + cos(psi)*sin(theta)*cos(phi);
     sin(psi)*cos(theta), cos(psi)*cos(phi) + sin(psi)*sin(theta)*sin(phi), -cos(psi)*sin(phi) + sin(psi)*sin(theta)*cos(phi);
     -sin(theta), cos(theta)*sin(phi), cos(theta)*cos(phi)];

E_B = [-b*sin(alpha), -b*sin(alpha), -b*sin(beta), -b*sin(beta);
        0,0,0,0;
        -b*cos(alpha), -b*cos(alpha), -b*cos(beta), -b*cos(beta);
        b*l_l*cos(alpha) + d*sin(alpha), -1*(b*l_l*cos(alpha) + d*sin(alpha)), b*l_l*cos(beta) - d*sin(beta), -1*(b*l_l*cos(beta) - d*sin(beta));
        b*l_s*cos(alpha), b*l_s*cos(alpha), -1*(b*l_s)*cos(beta), -1*(b*l_s)*cos(beta);
        -b*l_l*sin(alpha) + d*cos(alpha), b*l_l*sin(alpha) - d*cos(alpha), -b*l_l*sin(beta) - d*cos(beta), b*l_l*sin(beta) + d*cos(beta)];
       
T = [R, zeros(3,3);
    zeros(3,3), eye(3)];


out = T*E_B;

== matlab function tilt_rotor_drone_controller/Quad Model Matrix/MATLAB Function3 ==
  data: mass input; out output; inertia input
function out = M_H(mass, inertia)

M = mass * eye(3);

out = [M, zeros(3,3);
    zeros(3,3), inertia];

== matlab function tilt_rotor_drone_controller/Quad Model Matrix/MATLAB Function4 ==
  data: s_dot input; out output size=[6,6]; inertia input
function out = C_H(s_dot, inertia)

skew = inertia*s_dot(4:6);

out = [zeros(3,3), zeros(3,3);
       zeros(1,3), 0, -skew(3), skew(2);
       zeros(1,3), skew(3), 0, -skew(1);
       zeros(1,3), -skew(2), skew(1), 0];

== matlab function tilt_rotor_drone_controller/Quad Model Matrix/MATLAB Function5 ==
  data: A input; inv_A output
function inv_A = m_inverse(A)
inv_A = inv(A);

== matlab function tilt_rotor_drone_controller/MATLAB Function ==
  data: s input; U output; s_d input; m input; I input; J_TP input; Q input; R input
function U = LQR(s, s_d, m, I, J_TP, Q, R)
% s_d = [x_d, 0, y_d, 0, z_d, 0, 0, 0, 0, 0, psi_d, 0]

coder.extrinsic('lqr');

Ix = I(1);
Iy = I(5);
Iz = I(9);

x = s(1);
y = s(3);
z = s(5);
psi = s(11);

theta = 0;
phi = 0;
q = 0;
r = 0;
p = 0;

g = 9.8;

U1 = m*g;
U2 = 0;
U3 = 0;
U4 = 0;
Omega = 0;

U_ss = [U1; U2; U3; U4; Omega];

A = [ 0, 1, 0, 0, 0, 0,                                                          0,       0,                                   0,        0,                                                         0, 0;
    0, 0, 0, 0, 0, 0,  (U1*(cos(phi)*sin(psi) - cos(psi)*sin(phi)*sin(theta)))/5,       0, (U1*cos(phi)*cos(psi)*cos(theta))/5,        0, (U1*(cos(psi)*sin(phi) - cos(phi)*sin(psi)*sin(theta)))/5, 0;
    0, 0, 0, 1, 0, 0,                                                          0,       0,                                   0,        0,                                                         0, 0;
    0, 0, 0, 0, 0, 0, -(U1*(cos(phi)*cos(psi) + sin(phi)*sin(psi)*sin(theta)))/5,       0, (U1*cos(phi)*cos(theta)*sin(psi))/5,        0, (U1*(sin(phi)*sin(psi) + cos(phi)*cos(psi)*sin(theta)))/5, 0;
    0, 0, 0, 0, 0, 1,                                                          0,       0,                                   0,        0,                                                         0, 0;
    0, 0, 0, 0, 0, 0,                                -(U1*cos(theta)*sin(phi))/5,       0,         -(U1*cos(phi)*sin(theta))/5,        0,                                                         0, 0;
    0, 0, 0, 0, 0, 0,                                                          0,       1,                                   0,        0,                                                         0, 0;
    0, 0, 0, 0, 0, 0,                                                          0,       0,                                   0, -5*Omega,                                                         0, 0;
    0, 0, 0, 0, 0, 0,                                                          0,       0,                                   0,        1,                                                         0, 0;
    0, 0, 0, 0, 0, 0,                                                          0, 5*Omega,                                   0,        0,                                                         0, 0;
    0, 0, 0, 0, 0, 0,                                                          0,       0,                                   0,        0,                                                         0, 1;
    0, 0, 0, 0, 0, 0,                                                          0,       0,                                   0,        0,                                                         0, 0];

% a1 = ((Iy-Iz)/Ix)*r - J_TP/Ix*Omega;
% a2 = ((Iz-Ix)/Iy)*r + J_TP/Iy*Omega;
% a3 = ((Ix-Iy)/Iz)*q;
% 
% A = [0,1,0,0,0,0,0,0,0,0,0,0;
%      0,0,0,0,0,0,0,0,0,0,0,0;
%      0,0,0,1,0,0,0,0,0,0,0,0;
%      0,0,0,0,0,0,0,0,0,0,0,0;
%      0,0,0,0,0,1,0,0,0,0,0,0;
%      0,0,0,0,0,0,0,0,0,0,0,0;
%      0,0,0,0,0,0,0,1,0,0,0,0;
%      0,0,0,0,0,0,0,0,0,a1,0,0;
%      0,0,0,0,0,0,0,0,0,1,0,0;
%      0,0,0,0,0,0,0,a2,0,0,0,0;
%      0,0,0,0,0,0,0,0,0,0,0,1;
%      0,0,0,0,0,0,0,a3,0,0,0,0];
 
B = [0,  0,  0,  0,    0;
    (sin(phi)*sin(psi))/5 + (cos(phi)*cos(psi)*sin(theta))/5,  0,  0,  0,    0;
    0,  0,  0,  0,    0;
    (cos(phi)*sin(psi)*sin(theta))/5 - (cos(psi)*sin(phi))/5,  0,  0,  0,    0;
    0,  0,  0,  0,    0;
    (cos(phi)*cos(theta))/5,  0,  0,  0,    0;
    0,  0,  0,  0,    0;
    0, 10,  0,  0, -5*q;
    0,  0,  0,  0,    0;
    0,  0, 10,  0,  5*p;
    0,  0,  0,  0,    0;
    0,  0,  0, 10,    0];

% b1 = (sin(psi)*sin(phi) + cos(psi)*sin(theta)*cos(phi))/m;
% b2 = (-cos(psi)*sin(phi) + sin(psi)*sin(theta)*cos(phi))/m;
% b3 = (cos(theta)*cos(phi))/m;
% b4 = 1/Ix;
% b5 = 1/Iy;
% b6 = 1/Iz;
% 
% B = [0,0,0,0,0;
%      b1,0,0,0,0;
%      0,0,0,0,0;
%      b2,0,0,0,0;
%      0,0,0,0,0;
%      b3,0,0,0,0;
%      0,0,0,0,0;
%      0,b4,0,0,0;
%      0,0,0,0,0;
%      0,0,b5,0,0;
%      0,0,0,0,0;
%      0,0,0,0,b6];

K = zeros(5,12);

[K,S,e] = lqr(A, B, Q, R);

ds = s_d - s;

U = U_ss - K*ds;

== matlab function tilt_rotor_drone_controller/Quad Mode Controller/MATLAB Function1 ==
  data: s input; U input size=4; l_s input; omega_1 output; omega_2 output; omega_3 output; omega_4 output; l_l input; lambda input; m input
function [omega_1, omega_2, omega_3, omega_4] = U_to_Omega(s, U, l_s, l_l, lambda, m)

% s = [x, dx, y, dy, z, dz, phi, p, theta, q, psi, r]
% U = [U2, U3, U4, Ux, Uy, Uz]
% U1 = b*(omega_1^2 + omega_2^2 + omega_3^2 + omega_4^2)
% U2 = lb*(-omega_2^2 + omega_4^2)
% U3 = lb*(-omega_1^2 + omega_3^2)
% U4 = d*(-omega_1^2 + omega_2^2 - omega_3^2 + omega_4^2)
% Ux = cos(phi)sin(theta)cos(psi) + sin(phi)cos(psi)
% Uy = cos(phi)sin(theta)sin(psi) - sin(phi)cos(psi)
% Uz = g + (cos(phi)cos(theta))*1/m*U1


phi = s(7);
theta = s(9);

g = 9.8;

U1 = m*(U(4) - g)/(cos(phi)*cos(theta));
% U1 = -(m*g)/(cos(phi)*cos(theta));

U_n = U(1:3);
U_n = [U1; U_n];

A = [-1, -1, -1, -1;
     l_s, -l_s, l_s, -l_s;
     l_l, l_l, -l_l, -l_l;
     lambda, -lambda, -lambda, lambda];

O_sqr = A\U_n;

if (O_sqr(1) > 0)
    omega_1 = sqrt(O_sqr(1));
else
    omega_1 = 0;
end

if (O_sqr(2) > 0)
    omega_2 = sqrt(O_sqr(2));
else
    omega_2 = 0;
end

if (O_sqr(3) > 0)
    omega_3 = sqrt(O_sqr(3));
else
    omega_3 = 0;
end

if (O_sqr(4) > 0)
    omega_4 = sqrt(O_sqr(4));
else
    omega_4 = 0;
end
